simulink model "VD_Model"  (R2023b)
settings: Solver=VariableStepAuto  StartTime=0.0  StopTime=10.0  RelTol=1e-3
settings Model: Creator=bglen  LastModifiedBy=bglen

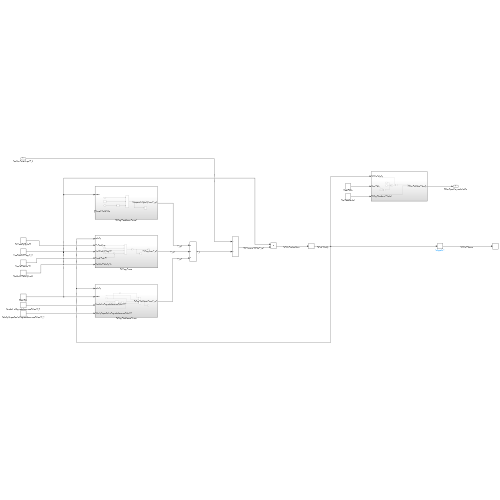
[thumbnail: Simulink's stored preview of the top-level diagram]
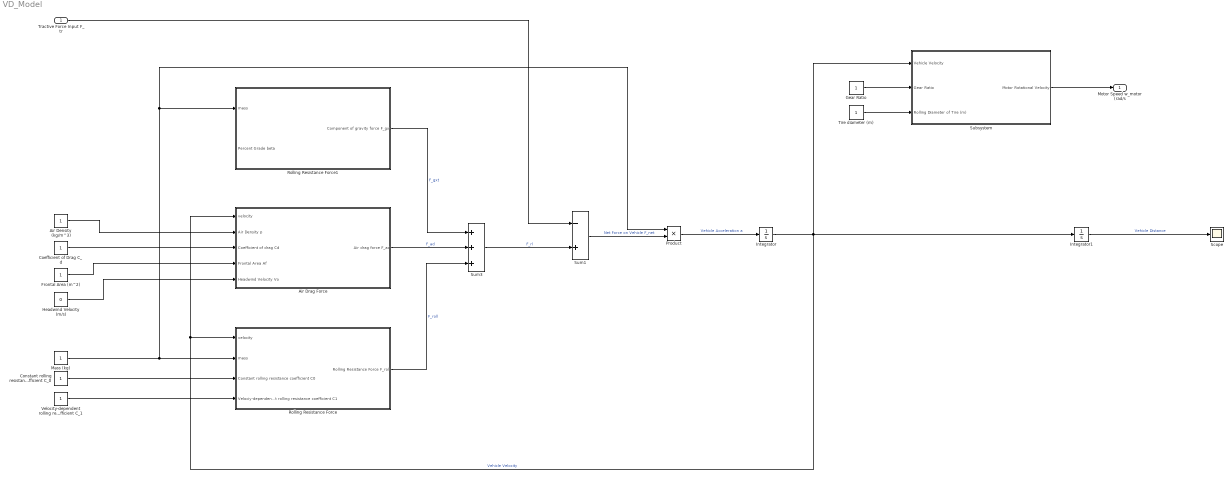
== system VD_Model ==
  Tractive Force Input F_tr : Inport
  Air Density (kg/m^3) : Constant
  "Air Drag Force " : Subsystem
  Coefficient of Drag C_d : Constant
  Constant rolling resistance coefficient C_0 : Constant
  Frontal Area (m^2) : Constant
  Gear Ratio : Constant
  Headwind Velocity (m/s) : Constant  Value=0
  Integrator : Integrator
  Integrator1 : Integrator
  Mass (kg) : Constant
  Product : Product
  Rolling Resistance Force : Subsystem
  Rolling Resistance Force1 : Subsystem
  Scope : Scope
  Subsystem : Subsystem
  Sum1 : Sum  Inputs=-+
  Sum3 : Sum  Inputs=+++
  Tire diameter (m) : Constant
  Velocity-dependent rolling resistance coefficient C_1 : Constant
  Motor Speed w_motor (rad/s : Outport
  wires:
  Mass (kg)/1 -> Product/1, Rolling Resistance Force1/1(mass), Rolling Resistance Force/2(mass)
  Constant rolling resistance coefficient C_0/1 -> Rolling Resistance Force/3(Constant rolling resistance coefficient C0)
  Velocity-dependent rolling resistance coefficient C_1/1 -> Rolling Resistance Force/4(Velociy-dependent rolling resistance coefficient C1)
  Air Density (kg/m^3)/1 -> "Air Drag Force "/2(Air Density p)
  Coefficient of Drag C_d/1 -> "Air Drag Force "/3(Coefficient of drag Cd)
  Frontal Area (m^2)/1 -> "Air Drag Force "/4(Frontal Area Af)
  Headwind Velocity (m/s)/1 -> "Air Drag Force "/5(Headwind Velocity Vo)
  "Air Drag Force "/1(Air drag force F_ad) -> Sum3/2  "F_ad"
  Rolling Resistance Force1/1(Component of gravity force F_gxt) -> Sum3/1  "F_gxt"
  Rolling Resistance Force/1(Rolling Resistance Force F_roll) -> Sum3/3  "F_roll"
  Sum1/1 -> Product/2  "Net Force on Vehicle F_net"
  Sum3/1 -> Sum1/2  "F_rl"
  Tractive Force Input F_tr/1 -> Sum1/1
  Product/1 -> Integrator/1  "Vehicle Acceleration a"
  Integrator/1 -> Integrator1/1, Subsystem/1(Vehicle Velocity), "Air Drag Force "/1(velocity), Rolling Resistance Force/1(velocity)  "Vehicle Velocity"
  Integrator1/1 -> Scope/1  "Vehicle Distance"
  Gear Ratio/1 -> Subsystem/2(Gear Ratio)
  Tire diameter (m)/1 -> Subsystem/3(Rolling Diameter of Tire (m))
  Subsystem/1(Motor Rotational Velocity) -> Motor Speed w_motor (rad/s/1

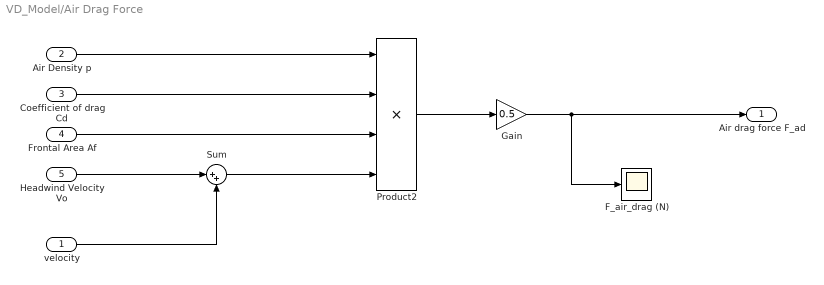
== system VD_Model/Air Drag Force  ==
  velocity : Inport
  Air Density p : Inport  Port=2
  Coefficient of drag Cd : Inport  Port=3
  Frontal Area Af : Inport  Port=4
  Headwind Velocity Vo : Inport  Port=5
  F_air_drag (N) : Scope
  Gain : Gain  Gain=0.5
  Product2 : Product  Inputs=4
  Sum : Sum  Inputs=|++
  Air drag force F_ad : Outport
  wires:
  velocity/1 -> Sum/2
  Air Density p/1 -> Product2/1
  Frontal Area Af/1 -> Product2/3
  Sum/1 -> Product2/4
  Gain/1 -> Air drag force F_ad/1, F_air_drag (N)/1
  Coefficient of drag Cd/1 -> Product2/2
  Headwind Velocity Vo/1 -> Sum/1
  Product2/1 -> Gain/1

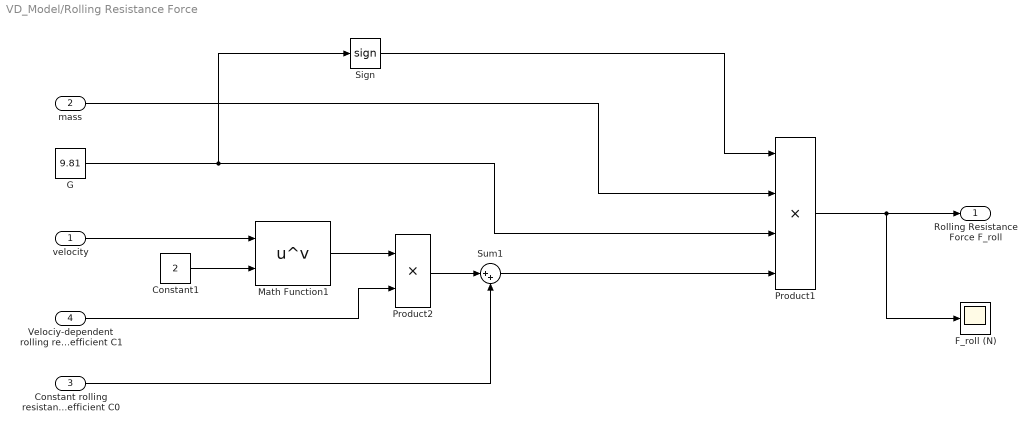
== system VD_Model/Rolling Resistance Force ==
  velocity : Inport
  mass : Inport  Port=2
  Constant rolling resistance coefficient C0 : Inport  Port=3
  Velociy-dependent rolling resistance coefficient C1 : Inport  Port=4
  Constant1 : Constant  Value=2
  F_roll (N) : Scope
  G : Constant  Value=9.81
  Math Function1 : Math  Operator=pow
  Product1 : Product  Inputs=4
  Product2 : Product
  Sign : Signum
  Sum1 : Sum  Inputs=|++
  Rolling Resistance Force F_roll : Outport
  wires:
  Sum1/1 -> Product1/4
  velocity/1 -> Math Function1/1
  Product1/1 -> F_roll (N)/1, Rolling Resistance Force F_roll/1
  Constant1/1 -> Math Function1/2
  Constant rolling resistance coefficient C0/1 -> Sum1/2
  Velociy-dependent rolling resistance coefficient C1/1 -> Product2/2
  Math Function1/1 -> Product2/1
  Product2/1 -> Sum1/1
  mass/1 -> Product1/2
  Sign/1 -> Product1/1
  G/1 -> Product1/3, Sign/1

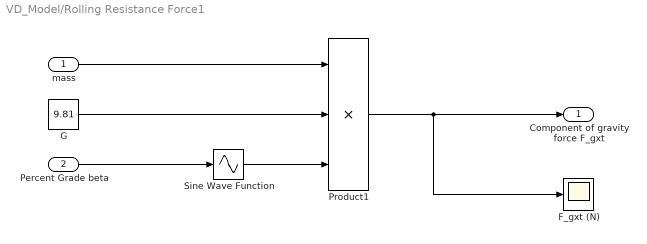
== system VD_Model/Rolling Resistance Force1 ==
  mass : Inport
  Percent Grade beta : Inport  Port=2
  F_gxt (N) : Scope
  G : Constant  Value=9.81
  Product1 : Product  Inputs=3
  Sine Wave Function : Sin  TimeSource=Use external signal  SampleTime=0
  Component of gravity force F_gxt : Outport
  wires:
  Product1/1 -> Component of gravity force F_gxt/1, F_gxt (N)/1
  mass/1 -> Product1/1
  G/1 -> Product1/2
  Percent Grade beta/1 -> Sine Wave Function/1
  Sine Wave Function/1 -> Product1/3

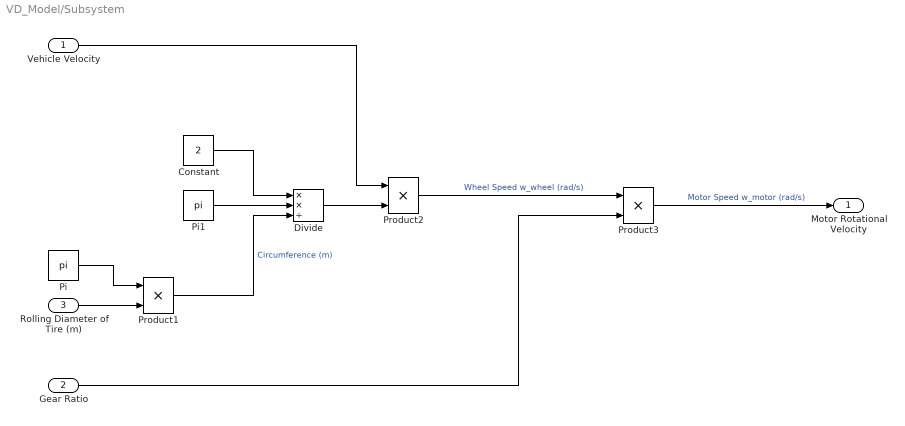
== system VD_Model/Subsystem ==
  Vehicle Velocity : Inport
  Gear Ratio : Inport  Port=2
  Rolling Diameter of Tire (m) : Inport  Port=3
  Constant : Constant  Value=2
  Divide : Product  Inputs=**/
  Pi : Constant  Value=pi  OutDataTypeStr=Inherit: Inherit via back propagation
  Pi1 : Constant  Value=pi  OutDataTypeStr=Inherit: Inherit via back propagation
  Product1 : Product
  Product2 : Product
  Product3 : Product
  Motor Rotational Velocity : Outport
  wires:
  Pi/1 -> Product1/1
  Rolling Diameter of Tire (m)/1 -> Product1/2
  Constant/1 -> Divide/1
  Pi1/1 -> Divide/2
  Product1/1 -> Divide/3  "Circumference (m)"
  Vehicle Velocity/1 -> Product2/1
  Divide/1 -> Product2/2
  Product2/1 -> Product3/1  "Wheel Speed w_wheel (rad/s)"
  Gear Ratio/1 -> Product3/2
  Product3/1 -> Motor Rotational Velocity/1  "Motor Speed w_motor (rad/s)"
